simulink model "RealGrid"  (R2015b)
settings: Solver=VariableStepAuto  StartTime=0.0  StopTime=10.0  RelTol=1e-3
libraries: powerlib x9, powerlib_meascontrol x2
settings Model: Creator=Emilio  LastModifiedBy=Emilio

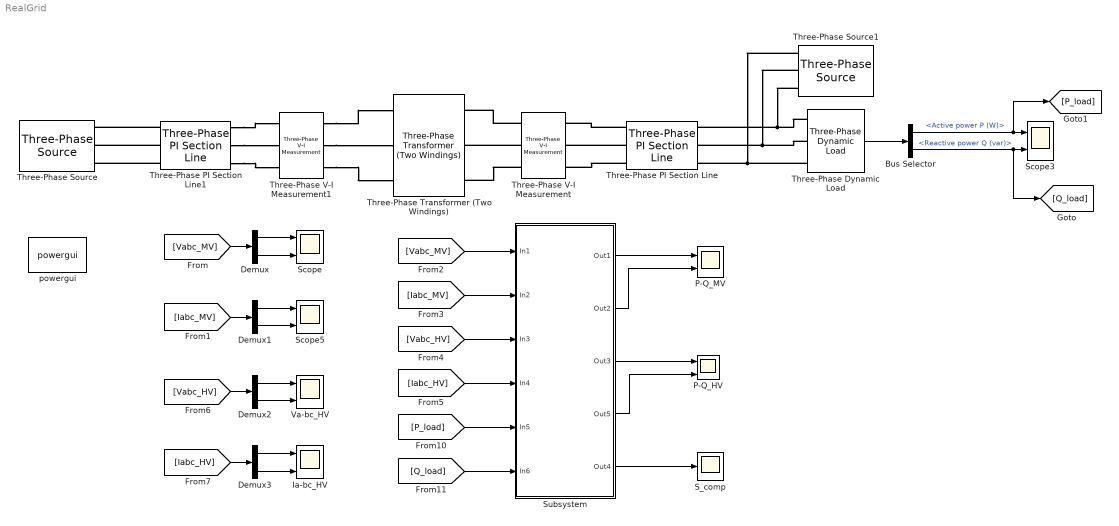
== system RealGrid ==
  Bus Selector : BusSelector  OutputSignals=Active power P (W),Reactive power Q (var)
  Demux{,1..3} (4 alike) : Demux  Outputs=[1 2]
  Ia-bc_HV : Scope  NumInputPorts=2
  P-Q_HV : Scope  NumInputPorts=2
  P-Q_MV : Scope  NumInputPorts=2
  S_comp : Scope
  Scope : Scope  NumInputPorts=2
  Scope3 : Scope  NumInputPorts=2
  Scope5 : Scope  NumInputPorts=2
  Subsystem : Subsystem
  Three-Phase Dynamic Load : powerlib/Elements/Three-Phase Dynamic Load  NominalVoltage=[ 400e3 50]  ActiveReactivePowers=[50e6 25e6]  PositiveSequence=[0.994 -11.8]  ExternalControl=off  NpNq=[1.3 2]  TimeConstants="[0.25  0.5  0.25  0.3]"  MinimumVoltage=0.7  LoadFlowParameters=[4,0,0,0,0]
  Three-Phase PI Section Line : powerlib/Elements/Three-Phase PI Section Line  LConnTagsString=a|b|c  RConnTagsString=A|B|C  Frequency=50  Resistances=[ 0.01273 0.3864]  Inductances="[ 0.9337e-3  4.1264e-3]"  Capacitances=[12.74e-9 7.751e-9]  Length=100
  Three-Phase PI Section Line1 : powerlib/Elements/Three-Phase PI Section Line  LConnTagsString=a|b|c  RConnTagsString=A|B|C  Frequency=50  Resistances=[ 0.01273 0.3864]  Inductances="[ 0.9337e-3  4.1264e-3]"  Capacitances=[12.74e-9 7.751e-9]  Length=20
  Three-Phase Transformer (Two Windings) : powerlib/Elements/Three-Phase Transformer (Two Windings)  Winding1Connection=Yg  Winding2Connection=Yg  CoreType=Three single-phase transformers  SetSaturation=off  Hysteresis=off  DataFile='hysteresis'  SetInitialFlux=off  Measurements=None  UNITS=pu  NominalPower=[ 100e3 , 50 ]  Winding1=[ 220e3 , 0.002 , 0.08 ]  Winding2=[ 400e3 , 0.002 , 0.08 ]  Rm=500  Lm=500  L0=0.50001  Saturation=[ 0,0 ; 0.0024,1.2 ; 1.0,1.52 ]  InitialFluxes=[ 0.8 , -0.8 , 0.7 ]  MoreParameters=off  BreakLoop=off  DataType=off  TransfoNumber=1
  Three-Phase V-I Measurement : powerlib/Measurements/Three-Phase V-I Measurement  VoltageMeasurement=phase-to-ground  SetLabelV=on  LabelV=Vabc_HV  Vpu=off  VpuLL=off  CurrentMeasurement=yes  SetLabelI=on  LabelI=Iabc_HV  Ipu=off  Pbase=100e6  Vbase=500e3  OutputType=Complex  PhasorSimulation=on  PSBequivalent=0
  Three-Phase V-I Measurement1 : powerlib/Measurements/Three-Phase V-I Measurement  VoltageMeasurement=phase-to-ground  SetLabelV=on  LabelV=Vabc_MV  Vpu=off  VpuLL=off  CurrentMeasurement=yes  SetLabelI=on  LabelI=Iabc_MV  Ipu=off  Pbase=100e6  Vbase=500e3  OutputType=Complex  PhasorSimulation=on  PSBequivalent=0
  Three-Phase Source : powerlib/Electrical Sources/Three-Phase Source  InternalConnection=Yg  VoltagePhases=off  Voltage=220e3  PhaseAngle=0  Voltage_phases=[25e3 25e3 25e3]/sqrt(3)  PhaseAngles_phases=[0 -120 +120]  Frequency=50  NonIdealSource=on  SpecifyImpedance=off  Resistance=0.8929  Inductance=16.58e-3  ShortCircuitLevel=100e6  BaseVoltage=25e3  XRratio=7  BusType=PQ  Pref=10e3  Qref=0  Prefabc=[10e3, 10e3, 10e3]  Qrefabc=[0, 0, 0]  Qmin=-inf  Qmax=inf
  Three-Phase Source1 : powerlib/Electrical Sources/Three-Phase Source  InternalConnection=Yg  VoltagePhases=off  Voltage=400e3  PhaseAngle=0  Voltage_phases=[25e3 25e3 25e3]/sqrt(3)  PhaseAngles_phases=[0 -120 +120]  Frequency=50  NonIdealSource=on  SpecifyImpedance=off  Resistance=0.8929  Inductance=16.58e-3  ShortCircuitLevel=100e6  BaseVoltage=25e3  XRratio=7  BusType=swing  Pref=10e3  Qref=0  Prefabc=[10e3, 10e3, 10e3]  Qrefabc=[0, 0, 0]  Qmin=-inf  Qmax=inf
  Va-bc_HV : Scope  NumInputPorts=2
  powergui : powerlib/powergui  Priority=1  SimulationMode=Phasor  SolverType=Tustin/Backward Euler (TBE)  SampleTime=50e-6  frequency=50  SPID=off  DisableSnubberDevices=off  DisableRonSwitches=off  DisableVfSwitches=off  SwTol=0  DisplayEquations=off  Interpol=off  ExternalGateDelay=off  methode=off  Ts=10  FunctionMessages=off  echomessages=off  HookPort=off  EnableUseOfTLC=off  x0status=blocks  frequencyindice=50  Pbase=100e6  ErrMax=1e-4  Iterations=50  UnitsV=V  UnitsW=W  buscounter=0  RestoreLinks=warning  ResistiveCurrentMeasurement=off  Frange=[0:2:500]  Ylog=off  Xlog=on  ShowGrid=off  save=off  variable=ZData  structure=0  ZoomFFT=off  StartTime=0.0  cycles=1  DisplayStyle=1  fundamental=60  FreqAxis=off  MaxFrequency=1000  frequencyindicesteady=1  RmsSteady=1  display=off
  wires:
  Bus Selector/1 -> [P_load], Scope3/1  "<Active power P (W)>"
  Bus Selector/2 -> [Q_load], Scope3/2  "<Reactive power Q (var)>"
  Three-Phase Dynamic Load/1 -> Bus Selector/1
  [Vabc_MV] -> Demux/1
  Demux/1 -> Scope/1
  Demux/2 -> Scope/2
  [Iabc_MV] -> Demux1/1
  Demux1/1 -> Scope5/1
  Demux1/2 -> Scope5/2
  [Vabc_MV] -> Subsystem/1(In1)
  [Iabc_MV] -> Subsystem/2(In2)
  [Vabc_HV] -> Subsystem/3(In3)
  [Iabc_HV] -> Subsystem/4(In4)
  [P_load] -> Subsystem/5(In5)
  [Q_load] -> Subsystem/6(In6)
  Subsystem/1(Out1) -> P-Q_MV/1
  Subsystem/2(Out2) -> P-Q_MV/2
  Subsystem/3(Out3) -> P-Q_HV/1
  Subsystem/5(Out4) -> S_comp/1
  Subsystem/4(Out5) -> P-Q_HV/2
  Demux2/2 -> Va-bc_HV/2
  [Iabc_HV] -> Demux3/1
  Demux3/1 -> Ia-bc_HV/1
  Demux3/2 -> Ia-bc_HV/2
  Demux2/1 -> Va-bc_HV/1
  [Vabc_HV] -> Demux2/1
  connections:
  Three-Phase PI Section Line/LConn3 -- Three-Phase V-I Measurement/RConn3
  Three-Phase V-I Measurement/LConn2 -- Three-Phase Transformer (Two Windings)/RConn2
  Three-Phase PI Section Line/LConn2 -- Three-Phase V-I Measurement/RConn2
  Three-Phase V-I Measurement/LConn1 -- Three-Phase Transformer (Two Windings)/RConn1
  Three-Phase PI Section Line1/LConn1 -- Three-Phase Source/RConn1
  Three-Phase PI Section Line1/LConn2 -- Three-Phase Source/RConn2
  Three-Phase V-I Measurement1/RConn3 -- Three-Phase Transformer (Two Windings)/LConn3
  Three-Phase PI Section Line1/LConn3 -- Three-Phase Source/RConn3
  Three-Phase PI Section Line1/RConn3 -- Three-Phase V-I Measurement1/LConn3
  Three-Phase V-I Measurement/LConn3 -- Three-Phase Transformer (Two Windings)/RConn3
  Three-Phase V-I Measurement1/RConn1 -- Three-Phase Transformer (Two Windings)/LConn1
  Three-Phase PI Section Line1/RConn1 -- Three-Phase V-I Measurement1/LConn1
  Three-Phase PI Section Line/LConn1 -- Three-Phase V-I Measurement/RConn1
  Three-Phase V-I Measurement1/RConn2 -- Three-Phase Transformer (Two Windings)/LConn2
  Three-Phase PI Section Line1/RConn2 -- Three-Phase V-I Measurement1/LConn2
  Three-Phase Dynamic Load/LConn1 -- Three-Phase Source1/RConn1 -- Three-Phase PI Section Line/RConn1
  Three-Phase Dynamic Load/LConn2 -- Three-Phase Source1/RConn2 -- Three-Phase PI Section Line/RConn2
  Three-Phase Dynamic Load/LConn3 -- Three-Phase Source1/RConn3 -- Three-Phase PI Section Line/RConn3

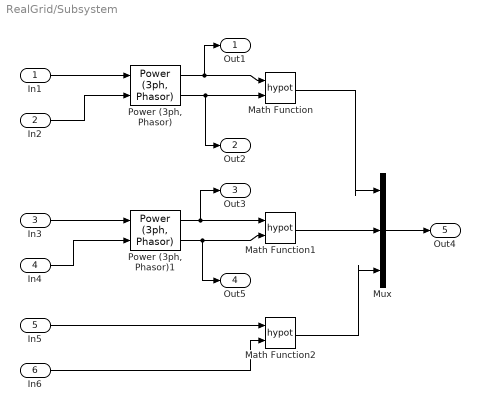
== system RealGrid/Subsystem ==
  In1 : Inport
  In2 : Inport  Port=2
  In3 : Inport  Port=3
  In4 : Inport  Port=4
  In5 : Inport  Port=5
  In6 : Inport  Port=6
  Math Function : Math  Operator=hypot  SaturateOnIntegerOverflow=on
  Math Function1 : Math  Operator=hypot  SaturateOnIntegerOverflow=on
  Math Function2 : Math  Operator=hypot  SaturateOnIntegerOverflow=on
  Mux : Mux  Inputs=3
  "Power (3ph, Phasor)" : powerlib_meascontrol/Measurements/Power (3ph, Phasor)
  "Power (3ph, Phasor)1" : powerlib_meascontrol/Measurements/Power (3ph, Phasor)
  Out1 : Outport
  Out2 : Outport  Port=2
  Out3 : Outport  Port=3
  Out5 : Outport  Port=4
  Out4 : Outport  Port=5
  wires:
  In6/1 -> Math Function2/2
  Mux/1 -> Out4/1
  "Power (3ph, Phasor)"/2 -> Out2/1, Math Function/2
  Math Function2/1 -> Mux/3
  "Power (3ph, Phasor)1"/2 -> Out5/1, Math Function1/2
  Math Function/1 -> Mux/1
  "Power (3ph, Phasor)1"/1 -> Out3/1, Math Function1/1
  Math Function1/1 -> Mux/2
  "Power (3ph, Phasor)"/1 -> Out1/1, Math Function/1
  In5/1 -> Math Function2/1
  In4/1 -> "Power (3ph, Phasor)1"/2
  In3/1 -> "Power (3ph, Phasor)1"/1
  In2/1 -> "Power (3ph, Phasor)"/2
  In1/1 -> "Power (3ph, Phasor)"/1
